simulink model "Practica10_CD"  (R2015a)
settings: Solver=ode45  StartTime=0.0  StopTime=100000  RelTol=1e-3
libraries: commchan3 x4, commutil2 x4, commsink2 x4, simulink x2, commrandsrc2 x1
settings Model: Creator=carlosfloresnava  LastModifiedBy=Isma

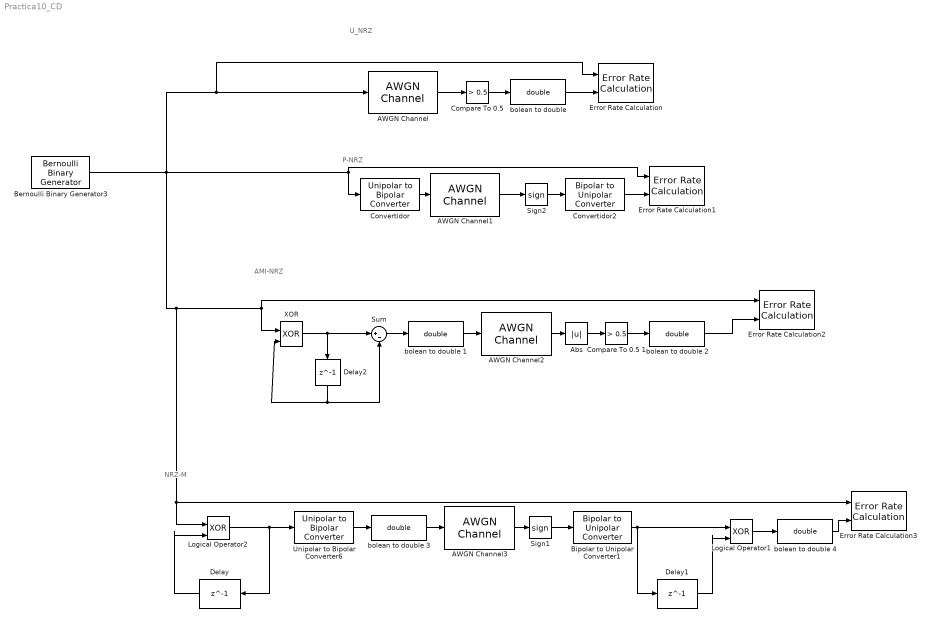
== system Practica10_CD ==
  note: NRZ-M
  note: AMI-NRZ
  note: P-NRZ
  note: U_NRZ
  AWGN Channel : commchan3/AWGN Channel  InputProcessing=Columns as channels (frame based)  seed=randseed  noiseMode="Signal to noise ratio  (Eb/No)"  EbNodB=x  EsNodB=10  SNRdB=10  bitsPerSym=1  Ps=0.5  Tsym=1  variance=10
  AWGN Channel1 : commchan3/AWGN Channel  InputProcessing=Columns as channels (frame based)  seed=randseed  noiseMode="Signal to noise ratio  (Eb/No)"  EbNodB=x  EsNodB=10  SNRdB=10  bitsPerSym=1  Ps=1  Tsym=1  variance=10
  AWGN Channel2 : commchan3/AWGN Channel  InputProcessing=Columns as channels (frame based)  seed=randseed  noiseMode="Signal to noise ratio  (Eb/No)"  EbNodB=x  EsNodB=10  SNRdB=10  bitsPerSym=1  Ps=1/2  Tsym=1  variance=10
  AWGN Channel3 : commchan3/AWGN Channel  InputProcessing=Columns as channels (frame based)  seed=randseed  noiseMode="Signal to noise ratio  (Eb/No)"  EbNodB=x  EsNodB=10  SNRdB=10  bitsPerSym=1  Ps=1  Tsym=1  variance=10
  Abs : Abs
  Bernoulli Binary Generator3 : commrandsrc2/Bernoulli Binary Generator  P=0.5  seed=randseed  Ts=1  frameBased=off  sampPerFrame=1  orient=off  outDataType=double
  Bipolar to Unipolar Converter1 : commutil2/Bipolar to Unipolar Converter  M=2  polarity=Positive  dataType=Same as input
  "Compare To 0.5 " : simulink/Logic and Bit Operations/Compare To Constant  relop=>  const=0.5  OutDataTypeStr=boolean
  Compare To 0.5 1 : simulink/Logic and Bit Operations/Compare To Constant  relop=>  const=0.5  OutDataTypeStr=boolean
  "Convertidor " : commutil2/Unipolar to Bipolar Converter  M=2  polarity=Positive  dataType=Inherit via internal rule
  Convertidor2 : commutil2/Bipolar to Unipolar Converter  M=2  polarity=Positive  dataType=Inherit via internal rule
  Delay : Delay  DelayLength=1  InitialCondition=0  InputProcessing=Inherited
  Delay1 : Delay  DelayLength=1  InitialCondition=0  InputProcessing=Inherited
  Delay2 : Delay  DelayLength=1  InitialCondition=0
  Error Rate Calculation : commsink2/Error Rate Calculation  N=0  st_delay=0  cp_mode=Entire frame  subframe=[]  PMode=Workspace  WsName=V_E1  RsMode2=off  stop=off  numErr=100  maxBits=1e6
  Error Rate Calculation1 : commsink2/Error Rate Calculation  N=0  st_delay=0  cp_mode=Entire frame  subframe=[]  PMode=Workspace  WsName=V_E2  RsMode2=off  stop=off  numErr=100  maxBits=1e6
  Error Rate Calculation2 : commsink2/Error Rate Calculation  N=0  st_delay=0  cp_mode=Entire frame  subframe=[]  PMode=Workspace  WsName=V_E3  RsMode2=off  stop=off  numErr=100  maxBits=1e6
  Error Rate Calculation3 : commsink2/Error Rate Calculation  N=0  st_delay=0  cp_mode=Entire frame  subframe=[]  PMode=Workspace  WsName=V_E4  RsMode2=off  stop=off  numErr=100  maxBits=1e6
  Logical Operator1 : Logic  Operator=XOR  IconShape=distinctive  AllPortsSameDT=off  OutDataTypeStr=boolean
  Logical Operator2 : Logic  Operator=XOR  IconShape=distinctive  AllPortsSameDT=off  OutDataTypeStr=boolean
  Sign1 : Signum
  Sign2 : Signum
  Sum : Sum  Inputs=|+-  OutDataTypeStr=double
  Unipolar to Bipolar Converter6 : commutil2/Unipolar to Bipolar Converter  M=2  polarity=Positive  dataType=Inherit via internal rule
  XOR : Logic  Operator=XOR  IconShape=distinctive  AllPortsSameDT=off  OutDataTypeStr=boolean
  bolean to double {,1..4} (5 alike) : DataTypeConversion  OutDataTypeStr=double
  wires:
  "bolean to double "/1 -> Error Rate Calculation/2
  "Compare To 0.5 "/1 -> "bolean to double "/1
  AWGN Channel/1 -> "Compare To 0.5 "/1
  Sign2/1 -> Convertidor2/1
  Convertidor2/1 -> Error Rate Calculation1/2
  AWGN Channel1/1 -> Sign2/1
  "Convertidor "/1 -> AWGN Channel1/1
  Delay2/1 -> Sum/2, XOR/2
  Sum/1 -> bolean to double 1/1
  Compare To 0.5 1/1 -> bolean to double 2/1
  XOR/1 -> Sum/1, Delay2/1
  bolean to double 2/1 -> Error Rate Calculation2/2
  bolean to double 1/1 -> AWGN Channel2/1
  Abs/1 -> Compare To 0.5 1/1
  AWGN Channel2/1 -> Abs/1
  Delay/1 -> Logical Operator2/2
  Logical Operator2/1 -> Unipolar to Bipolar Converter6/1, Delay/1
  bolean to double 4/1 -> Error Rate Calculation3/2
  bolean to double 3/1 -> AWGN Channel3/1
  Sign1/1 -> Bipolar to Unipolar Converter1/1
  Delay1/1 -> Logical Operator1/2
  Bipolar to Unipolar Converter1/1 -> Logical Operator1/1, Delay1/1
  Unipolar to Bipolar Converter6/1 -> bolean to double 3/1
  AWGN Channel3/1 -> Sign1/1
  Logical Operator1/1 -> bolean to double 4/1
  Bernoulli Binary Generator3/1 -> Error Rate Calculation/1, AWGN Channel/1, Logical Operator2/1, Error Rate Calculation3/1, XOR/1, Error Rate Calculation2/1, "Convertidor "/1, Error Rate Calculation1/1
